simulink library "calculateTargetWaypointReelIn_cl"  (R2018a)
settings: Solver=VariableStepAuto  StartTime=0.0  StopTime=10.0  RelTol=1e-3
undefined symbols (not defined in the file): ctrl
libraries: controllerComponents x3, lowLevel x2
settings Model: Creator=mitch  LastModifiedBy=mitch

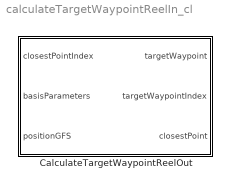
== system calculateTargetWaypointReelIn_cl ==
  CalculateTargetWaypointReelOut : Subsystem

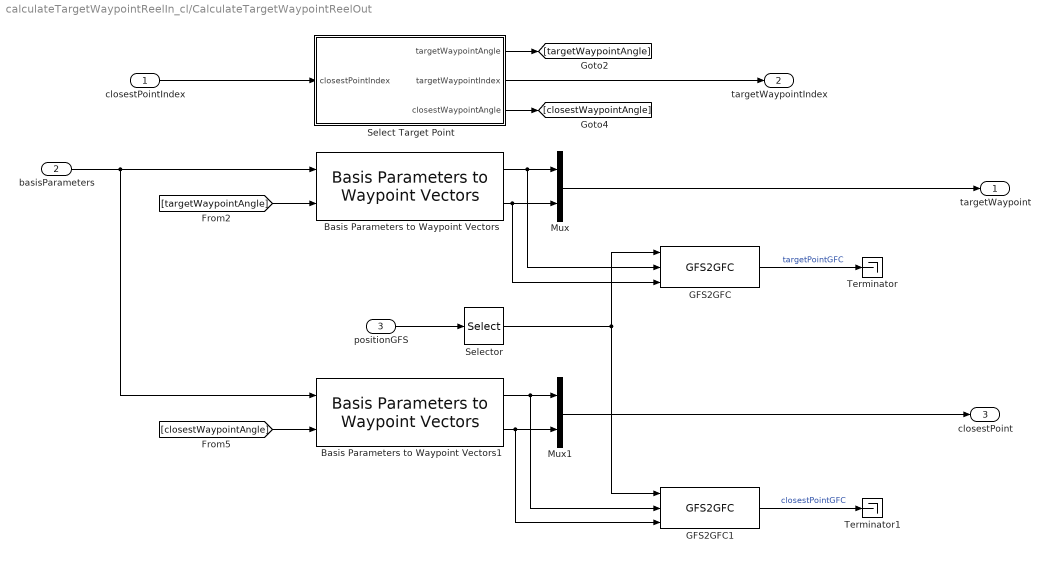
== system calculateTargetWaypointReelIn_cl/CalculateTargetWaypointReelOut ==
  closestPointIndex : Inport
  basisParameters : Inport  Port=2
  positionGFS : Inport  Port=3
  Basis Parameters to Waypoint Vectors : controllerComponents/Basis Parameters to Waypoint Vectors
  Basis Parameters to Waypoint Vectors1 : controllerComponents/Basis Parameters to Waypoint Vectors
  GFS2GFC : lowLevel/GFS2GFC
  GFS2GFC1 : lowLevel/GFS2GFC
  Mux : Mux  Inputs=2
  Mux1 : Mux  Inputs=2
  Select Target Point : Subsystem
  Selector : Selector  InputPortWidth=3  IndexOptions=Index vector (dialog)  Indices=1  OutputSizes=1
  Terminator : Terminator
  Terminator1 : Terminator
  targetWaypoint : Outport
  targetWaypointIndex : Outport  Port=2
  closestPoint : Outport  Port=3
  wires:
  GFS2GFC1/1 -> Terminator1/1  "closestPointGFC"
  Basis Parameters to Waypoint Vectors/2 -> GFS2GFC/3, Mux/2
  Select Target Point/3(closestWaypointAngle) -> [closestWaypointAngle]
  Select Target Point/1(targetWaypointAngle) -> [targetWaypointAngle]
  Mux1/1 -> closestPoint/1
  Basis Parameters to Waypoint Vectors/1 -> GFS2GFC/2, Mux/1
  [closestWaypointAngle] -> Basis Parameters to Waypoint Vectors1/2
  [targetWaypointAngle] -> Basis Parameters to Waypoint Vectors/2
  Basis Parameters to Waypoint Vectors1/2 -> GFS2GFC1/3, Mux1/2
  Basis Parameters to Waypoint Vectors1/1 -> GFS2GFC1/2, Mux1/1
  positionGFS/1 -> Selector/1
  closestPointIndex/1 -> Select Target Point/1(closestPointIndex)
  Mux/1 -> targetWaypoint/1
  Select Target Point/2(targetWaypointIndex) -> targetWaypointIndex/1
  GFS2GFC/1 -> Terminator/1  "targetPointGFC"
  basisParameters/1 -> Basis Parameters to Waypoint Vectors1/1, Basis Parameters to Waypoint Vectors/1
  Selector/1 -> GFS2GFC/1, GFS2GFC1/1

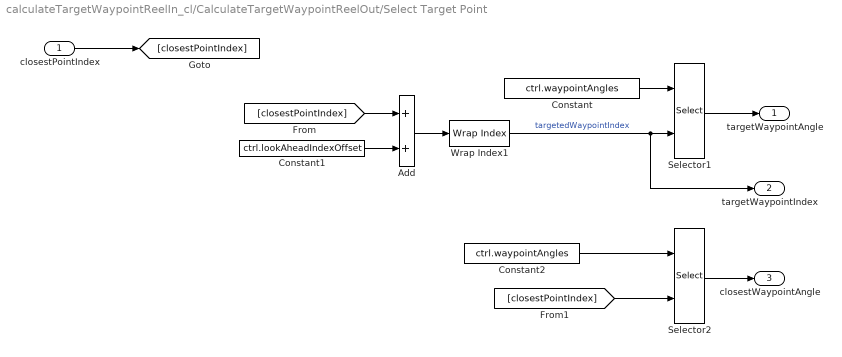
== system calculateTargetWaypointReelIn_cl/CalculateTargetWaypointReelOut/Select Target Point ==
  closestPointIndex : Inport
  Add : Sum
  Constant : Constant  Value=ctrl.waypointAngles
  Constant1 : Constant  Value=ctrl.lookAheadIndexOffset
  Constant2 : Constant  Value=ctrl.waypointAngles
  Selector1 : Selector  InputPortWidth=ctrl.num  IndexOptions=Index vector (port)  Indices=3  OutputSizes=1
  Selector2 : Selector  InputPortWidth=ctrl.num  IndexOptions=Index vector (port)  Indices=3  OutputSizes=1
  Wrap Index1 : controllerComponents/Wrap Index
  targetWaypointAngle : Outport
  targetWaypointIndex : Outport  Port=2
  closestWaypointAngle : Outport  Port=3
  wires:
  Constant/1 -> Selector1/1
  Constant1/1 -> Add/2
  Selector1/1 -> targetWaypointAngle/1
  Add/1 -> Wrap Index1/1
  Wrap Index1/1 -> targetWaypointIndex/1, Selector1/2  "targetedWaypointIndex"
  closestPointIndex/1 -> [closestPointIndex]
  [closestPointIndex] -> Add/1
  Constant2/1 -> Selector2/1
  [closestPointIndex] -> Selector2/2
  Selector2/1 -> closestWaypointAngle/1
